simulink library "HeatTransfer2Ground_ISO13370"  (R2018b)
settings: Solver=ode45  StartTime=0.0  StopTime=10.0  RelTol=1e-3  EnableMultiTasking=on
settings Model: Creator=drhf  LastModifiedBy=P41573
settings DataIOCC: LimitDataPoints=on  SaveFormat=Array  SignalLoggingSaveFormat=ModelDataLogs
settings OptimizationCC: ExpressionDepthLimit=2147483647  LifeSpan=inf
settings DebuggingCC: UnderspecifiedInitializationDetection=Classic  MergeDetectMultiDrivingBlocksExec=none  SolverPrmCheckMsg=warning  FcnCallInpInsideContextMsg=warning  StateNameClashWarn=warning  SFUnexpectedBacktrackingDiag=warning  SFNoUnconditionalDefaultTransitionDiag=warning  SFExecutionAtInitializationDiag=none
settings HardwareCC: ProdBitPerPointer=32  ProdBitPerSizeT=32  ProdBitPerPtrDiffT=32  ProdLargestAtomicFloat=None  ProdIntDivRoundTo=Undefined  ProdEndianess=Unspecified  ProdWordSize=32  ProdHWDeviceType=32-bit Generic
settings ModelReferenceCC: PropagateSignalLabelsOutOfModel=off
settings SFSimCC: SimUseLocalCustomCode=off
settings RTWCC: RTWUseLocalCustomCode=off
settings CodeAppCC: StateflowObjectComments=on
settings GRTTargetCC: TargetLangStandard=C89/C90 (ANSI)  GeneratePreprocessorConditionals=Disable all  CombineOutputUpdateFcns=off  GRTInterface=on
settings ConfigComp: CovMetricSettings=dw  CovHtmlReporting=on  CovSaveCumulativeToWorkspaceVar=on  CovSaveSingleToWorkspaceVar=on  CovExternalEMLEnable=off

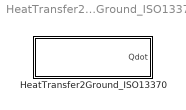
== system HeatTransfer2Ground_ISO13370 ==
  HeatTransfer2Ground_ISO13370 : Subsystem  mask(Heat Transfer to Ground ISO 13370){slabwidth=10, slablength=7, gammat=0, Tmeaninside=23.8, deltathetai=3.8, Tmeanoutside=11, deltathetae=9.3, tshift=319*3600, dwall=0.4, cond_ground=2.0, cp_ground=800, rho_ground=2500, utot=0.183}
      mask prompts: slabwidth "Width of slab in m"; slablength "Length of slab in m"; gammat "Linear thermal transmittance associated with wall/floor junctions [W/mK]"; Tmeaninside "Mean annual inside temperature [°C]"; deltathetai "Annual amplitude of inside temperature [°C]"; Tmeanoutside "Mean annual outside temperature [°C]"; deltathetae "Annual amplitude of outside temperature [°C]"; tshift "Time shift where outside temperature sine-curve shows a mimimum [s]"; dwall "Average thickness of walls inlcuding all layers [m]"; cond_ground "Conductivity of ground [W/(m*K)]"; cp_ground "Capacity of ground [J/(kg*K)]"; rho_ground "Density of ground [kg/m^3]"; utot "Total heat transfer of slab to ground [W/m²/K]"
      mask help:
      | Ground heat transfer for a floor "SLAB ON GROUND" according to ISO 13370:2007.
      | Use function fitSineToTamb to find the weather parameters.
      mask Help: web(fullfile(path_carnot('help'),'Heattransfer2GroundISO.html'),'-helpbrowser')
      mask Display: disp('U(ground)\nISO13370')

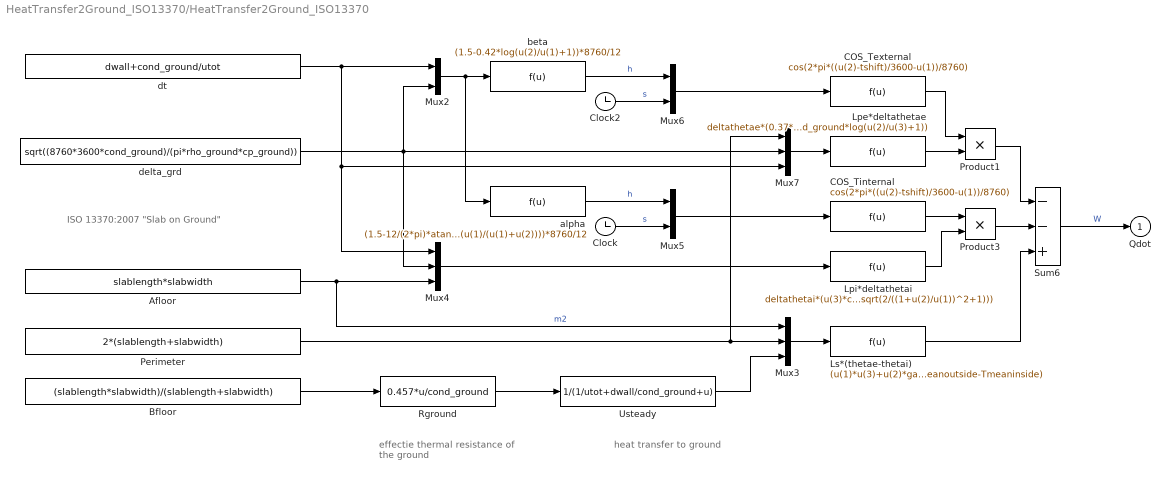
== system HeatTransfer2Ground_ISO13370/HeatTransfer2Ground_ISO13370 ==
  note: ISO 13370:2007 "Slab on Ground"
  note: effectie thermal resistance
      | of the ground
  note: heat transfer
      | to ground
  Afloor : Constant  Value=slablength*slabwidth
  Bfloor : Constant  Value=(slablength*slabwidth)/(slablength+slabwidth)
  COS_Texternal : Fcn  Expr=cos(2*pi*((u(2)-tshift)/3600-u(1))/8760)
  COS_Tinternal : Fcn  Expr=cos(2*pi*((u(2)-tshift)/3600-u(1))/8760)
  Clock : Clock
  Clock2 : Clock
  Lpe*deltathetae : Fcn  Expr=deltathetae*(0.37*u(1)*cond_ground*log(u(2)/u(3)+1))
  Lpi*deltathetai : Fcn  Expr=deltathetai*(u(3)*cond_ground/u(1)*sqrt(2/((1+u(2)/u(1))^2+1)))
  Ls*(thetae-thetai) : Fcn  Expr=(u(1)*u(3)+u(2)*gammat)*(Tmeanoutside-Tmeaninside)
  Mux2 : Mux  Inputs=2
  Mux3 : Mux  Inputs=3
  Mux4 : Mux  Inputs=3
  Mux5 : Mux  Inputs=2
  Mux6 : Mux  Inputs=2
  Mux7 : Mux  Inputs=3
  Perimeter : Constant  Value=2*(slablength+slabwidth)
  Product1 : Product  SaturateOnIntegerOverflow=on  RndMeth=Zero  InputSameDT=on  OutDataTypeStr=Inherit: Same as first input
  Product3 : Product  SaturateOnIntegerOverflow=on  RndMeth=Zero  InputSameDT=on  OutDataTypeStr=Inherit: Same as first input
  Rground : Fcn  Expr=0.457*u/cond_ground
  Sum6 : Sum  Inputs=--+
  Usteady : Fcn  Expr=1/(1/utot+dwall/cond_ground+u)
  alpha : Fcn  Expr=(1.5-12/(2*pi)*atan(u(1)/(u(1)+u(2))))*8760/12
  beta : Fcn  Expr=(1.5-0.42*log(u(2)/u(1)+1))*8760/12
  delta_grd : Constant  Value=sqrt((8760*3600*cond_ground)/(pi*rho_ground*cp_ground))
  dt : Constant  Value=dwall+cond_ground/utot
  Qdot : Outport
  wires:
  Sum6/1 -> Qdot/1  "W"
  Mux7/1 -> Lpe*deltathetae/1
  Product1/1 -> Sum6/1
  Lpe*deltathetae/1 -> Product1/2
  COS_Texternal/1 -> Product1/1
  Mux6/1 -> COS_Texternal/1
  Clock2/1 -> Mux6/2  "s"
  beta/1 -> Mux6/1  "h"
  Ls*(thetae-thetai)/1 -> Sum6/3
  Product3/1 -> Sum6/2
  COS_Tinternal/1 -> Product3/1
  Mux5/1 -> COS_Tinternal/1
  Clock/1 -> Mux5/2  "s"
  alpha/1 -> Mux5/1  "h"
  Lpi*deltathetai/1 -> Product3/2
  Mux4/1 -> Lpi*deltathetai/1
  Usteady/1 -> Mux3/3
  Perimeter/1 -> Mux7/1, Mux3/2
  Afloor/1 -> Mux3/1, Mux4/3  "m2"
  Mux3/1 -> Ls*(thetae-thetai)/1
  Mux2/1 -> beta/1, alpha/1
  delta_grd/1 -> Mux7/2, Mux4/2, Mux2/2
  dt/1 -> Mux2/1, Mux4/1, Mux7/3
  Bfloor/1 -> Rground/1
  Rground/1 -> Usteady/1
